simulink model "ThrottleArea"  (R2025b)
settings: Solver=VariableStepAuto  StartTime=0.0  StopTime=10.0  RelTol=1e-3
undefined symbols (not defined in the file or in its folder): alpha_0, alpha_1
settings Model: Creator=khanh  LastModifiedBy=khanh

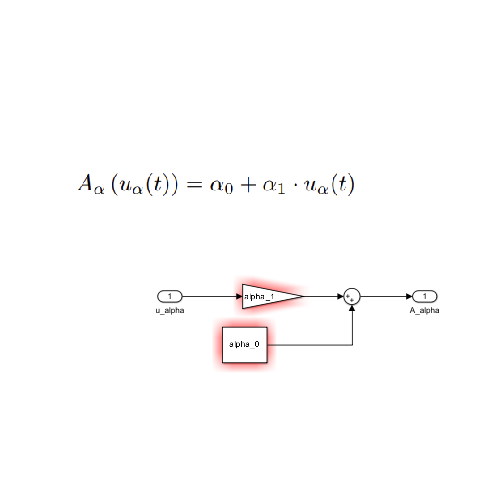
[thumbnail: Simulink's stored preview of the top-level diagram]
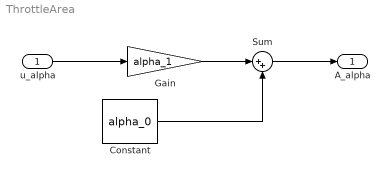
== system ThrottleArea ==
  u_alpha : Inport
  Constant : Constant  Value=alpha_0
  Gain : Gain  Gain=alpha_1
  Sum : Sum  Inputs=|++
  A_alpha : Outport
  wires:
  u_alpha/1 -> Gain/1
  Gain/1 -> Sum/1
  Constant/1 -> Sum/2
  Sum/1 -> A_alpha/1
